simulink model "digital_twin_model_v2"  (R2023a)
settings: Solver=FixedStepAuto  StartTime=0.0  StopTime=515  FixedStep=ts  RelTol=1e-3
values from neighbouring files (symbols this model uses):
  Ccell0 = cell0 / v_cell    (= 15384.6153846)    [MainCode.m]
  CG0 = 185    [MainCode.m]
  cg_noGrowth = 10    [MainCode.m]
  CM = 4    [MainCode.m]
  CO0 = .245    (= 0.245)    [MainCode.m]
  count_thresh = 3    [MainCode.m]
  F_fresh_start = 5 * .016 * 60    (= 4.8)    [MainCode.m]
  F_net = F_fresh_start + F_recycle_start    (= 334.8)    [MainCode.m]
  F_recycle_start = 5 * 1.1 * 60    (= 330)    [MainCode.m]
  freshPump_response_increases = 2    [MainCode.m]
  freshPump_response_window = 10    [MainCode.m]
  g_fault_wait_time = 10    [MainCode.m]
  g_flowrate_control_windowsize = 10    [MainCode.m]
  g_lownoise_val = 1.25    [MainCode.m]
  g_numpoints_fail = g_standdev_window_size+1    (= 16)    [MainCode.m]
  g_numpoints_low = 4    [MainCode.m]
  g_prob_arraylen = 15    [MainCode.m]
  g_prob_count = 6    [MainCode.m]
  g_prob_thresh = .45    (= 0.45)    [MainCode.m]
  g_standdev_window_size = 15    [MainCode.m]
  g_standev_tol = 7    [MainCode.m]
  mu_max = 0.0251    [MainCode.m]
  n_size = t_window/ts    (= 2.5)    [MainCode.m]
  n_size_CG = n_size    (= 2.5)    [MainCode.m]
  o2_fail_mean = .008    (= 0.008)    [MainCode.m]
  o2_fault_halfrange = .01    (= 0.01)    [MainCode.m]
  o2_fault_numpoints = 5    [MainCode.m]
  o2_lownoise_val = .0008    (= 0.0008)    [MainCode.m]
  o2_numpoints_low = 6    [MainCode.m]
  o2_prob_arraylen = 10    [MainCode.m]
  o2_prob_count = 6    [MainCode.m]
  o2_prob_thresh = .45    (= 0.45)    [MainCode.m]
  OCR = 2.8e-11    [MainCode.m]
  p_thresh = .4    (= 0.4)    [MainCode.m]
  recPump_drop_val = .02    (= 0.02)    [MainCode.m]
  recPump_rollingavg_samples_buildup = 10    [MainCode.m]
  recPump_smallDrop_size = 0.006    [MainCode.m]
  t_crit_CG = .7    (= 0.7)    [MainCode.m]
  ts = 1    [MainCode.m]
  V = 65.0    (= 65)    [MainCode.m]
  v_cell = 65    [MainCode.m]
  YGC = 155 * 10^-6    (= 0.000155)    [MainCode.m]
undefined symbols (not defined in the file or in its folder): DiscIntNeverNeededParam
libraries: simulink x10, sldrtlib x9, dspstat3 x6, aerolibanimutils x1
(part 1 of 2)
settings Model: Creator=axtaw  LastModifiedBy=axtaw
settings ModelReferenceCC: ModelReferenceMinAlgLoopOccurrences=on

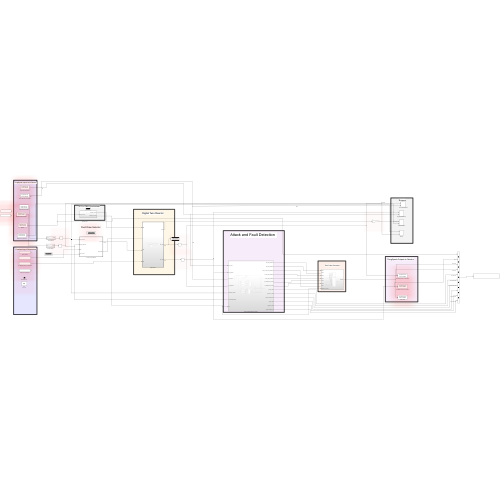
[thumbnail: Simulink's stored preview of the top-level diagram]
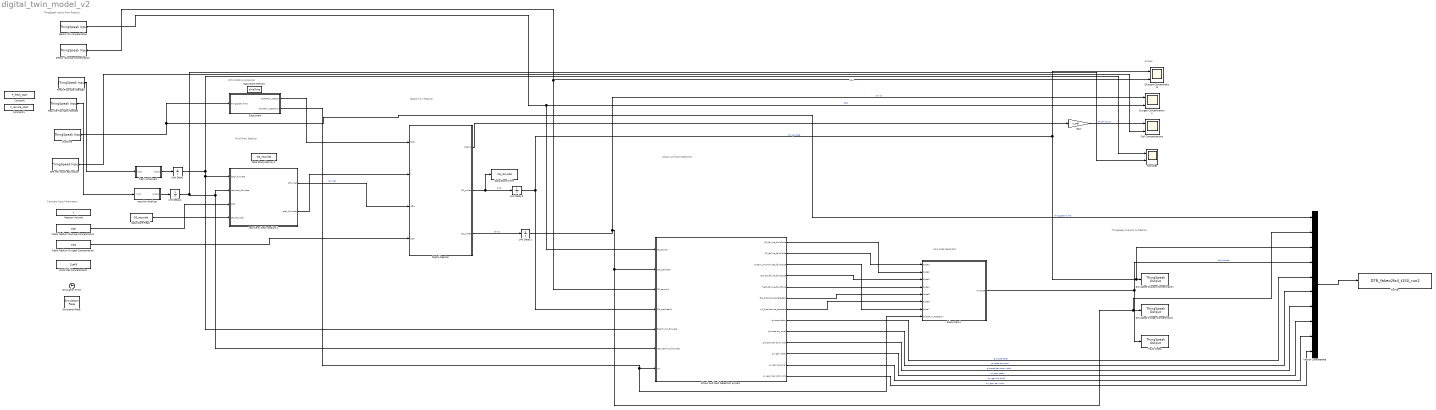
== system digital_twin_model_v2 ==
  note: Fluid Draw Selector
  note: DTR-CCBR Synchonizer
  note: Digital Twin Reactor
  note: Scopes
  note: Constant Input Parameters
  note: ThingSpeak Outputs to Reactor
  note: ThingSpeak Inputs from Reactor
  note: Attack and Fault Detection
  note: Faul Code Generator
  Attack and Fault Detection System : Subsystem
  Cell Concentrations : Scope  NumInputPorts=2
  Constant : Constant  Value=F_fresh_start
  Constant1 : Constant  Value=F_recycle_start
  Data Store Memory : DataStoreMemory  DataStoreName=aliveTime  WriteAfterWriteMsg=warning  ShowAdditionalParam=off
  Data Store Memory1 : DataStoreMemory  DataStoreName=CG_recycled  WriteAfterWriteMsg=warning  InitialValue=CG0  ShowAdditionalParam=off
  Data Store Read : DataStoreRead  DataStoreName=CG_recycled  IndexOptions=Index vector (dialog)  Indices=1  OutputSizes=1
  Data Store Write : DataStoreWrite  DataStoreName=CG_recycled  IndexOptions=Index vector (dialog)  Indices=1  OutputSizes=1
  Digital Reactor : Subsystem  TreatAsAtomicUnit=on
  Fault Codes : sldrtlib/Internet of Things/ThingSpeak Output  DrvAddress=2409205  DrvOptions=[1 1 50 75 54 78 55 57 69 50 79 79 81 55 79 66 88 72 97 112 105 46 116 104 105 110 103 115 112 101 97 107 46 99 111 109 0 0 0 0 0 0 0 0 0 0 0 0 0 0 0 0 0 0 0 0 0 0 0 0 0 0 0 0 0 0 0 0 0 0 0 0 0 0 0 0 0 0 0 0 0 0 0 0 0 0 0 0 0 0 0 0 0 0 0 0 0 0 0 0 0 0 0 0 0 0 0 0 0 0 0 0 0 0 0 0 0 0 0 0 0 0 0 0 0 0 0 0 0 0 0 0 0 0 0 0 0 0 0 0 0 0 0 0 0 0 0 0 0 0 0 0 0 0 0 0 0 0 0 0 0 0 0 0 0 0 0 0 0 0 0 0 0 0 0 0 0 0 0 0 0 0 0 0 0 0 0 0 0 0 0 0 0 0 0 0 0 0 0 0 0 0 0 0 0 0 0 0 0 0 0 0 0 0 0 0 0 0 0 0 0 0 0 0 0 0 0 0 0 0 0 0 0 0 0 0 0 0 0 0 0 0 0 0 0 0 0 0 0 0 0 0 0 0 0 0]  SampleTime=ts  MaxMissedTicks=1000  ShowMissedTicks=off  YieldWhenWaiting=off  ChannelFields=3  OptParam=0  InitialValue=[]  FinalValue=[]
  Fresh Flowrate Intended : sldrtlib/Internet of Things/ThingSpeak Input  DrvAddress=2409196  DrvOptions=[0 1 78 78 82 57 89 87 51 84 86 68 51 56 90 77 68 49 97 112 105 46 116 104 105 110 103 115 112 101 97 107 46 99 111 109 0 0 0 0 0 0 0 0 0 0 0 0 0 0 0 0 0 0 0 0 0 0 0 0 0 0 0 0 0 0 0 0 0 0 0 0 0 0 0 0 0 0 0 0 0 0 0 0 0 0 0 0 0 0 0 0 0 0 0 0 0 0 0 0 0 0 0 0 0 0 0 0 0 0 0 0 0 0 0 0 0 0 0 0 0 0 0 0 0 0 0 0 0 0 0 0 0 0 0 0 0 0 0 0 0 0 0 0 0 0 0 0 0 0 0 0 0 0 0 0 0 0 0 0 0 0 0 0 0 0 0 0 0 0 0 0 0 0 0 0 0 0 0 0 0 0 0 0 0 0 0 0 0 0 0 0 0 0 0 0 0 0 0 0 0 0 0 0 0 0 0 0 0 0 0 0 0 0 0 0 0 0 0 0 0 0 0 0 0 0 0 0 0 0 0 0 0 0 0 0 0 0 0 0 0 0 0 0 0 0 0 0 0 0 0 0 0 0 0 0]  SampleTime=ts  MaxMissedTicks=1000  ShowMissedTicks=off  YieldWhenWaiting=off  ChannelFields=3  OptParam=0  DataTypeStr=double
  Fresh Medium Glucose Concentration : Constant  Value=CG0
  Fresh Medium Oxygen Concentration : Constant  Value=CO0
  Gain : Gain  Gain=v_cell
  Glucose Concentrations : Scope  NumInputPorts=2
  Initial Cell Concentration : Constant  Value=Ccell0
  Oxygen Concentrations : Scope  NumInputPorts=2
  Reactor Volume : Constant  Value=V
  Recycle Flowrate Intended : sldrtlib/Internet of Things/ThingSpeak Input  DrvAddress=2409196  DrvOptions=[0 1 78 78 82 57 89 87 51 84 86 68 51 56 90 77 68 49 97 112 105 46 116 104 105 110 103 115 112 101 97 107 46 99 111 109 0 0 0 0 0 0 0 0 0 0 0 0 0 0 0 0 0 0 0 0 0 0 0 0 0 0 0 0 0 0 0 0 0 0 0 0 0 0 0 0 0 0 0 0 0 0 0 0 0 0 0 0 0 0 0 0 0 0 0 0 0 0 0 0 0 0 0 0 0 0 0 0 0 0 0 0 0 0 0 0 0 0 0 0 0 0 0 0 0 0 0 0 0 0 0 0 0 0 0 0 0 0 0 0 0 0 0 0 0 0 0 0 0 0 0 0 0 0 0 0 0 0 0 0 0 0 0 0 0 0 0 0 0 0 0 0 0 0 0 0 0 0 0 0 0 0 0 0 0 0 0 0 0 0 0 0 0 0 0 0 0 0 0 0 0 0 0 0 0 0 0 0 0 0 0 0 0 0 0 0 0 0 0 0 0 0 0 0 0 0 0 0 0 0 0 0 0 0 0 0 0 0 0 0 0 0 0 0 0 0 0 0 0 0 0 0 0 0 0 0]  SampleTime=ts  MaxMissedTicks=1000  ShowMissedTicks=off  YieldWhenWaiting=off  ChannelFields=2  OptParam=0  DataTypeStr=double
  Runtime : sldrtlib/Internet of Things/ThingSpeak Input  DrvAddress=2409196  DrvOptions=[0 1 78 78 82 57 89 87 51 84 86 68 51 56 90 77 68 49 97 112 105 46 116 104 105 110 103 115 112 101 97 107 46 99 111 109 0 0 0 0 0 0 0 0 0 0 0 0 0 0 0 0 0 0 0 0 0 0 0 0 0 0 0 0 0 0 0 0 0 0 0 0 0 0 0 0 0 0 0 0 0 0 0 0 0 0 0 0 0 0 0 0 0 0 0 0 0 0 0 0 0 0 0 0 0 0 0 0 0 0 0 0 0 0 0 0 0 0 0 0 0 0 0 0 0 0 0 0 0 0 0 0 0 0 0 0 0 0 0 0 0 0 0 0 0 0 0 0 0 0 0 0 0 0 0 0 0 0 0 0 0 0 0 0 0 0 0 0 0 0 0 0 0 0 0 0 0 0 0 0 0 0 0 0 0 0 0 0 0 0 0 0 0 0 0 0 0 0 0 0 0 0 0 0 0 0 0 0 0 0 0 0 0 0 0 0 0 0 0 0 0 0 0 0 0 0 0 0 0 0 0 0 0 0 0 0 0 0 0 0 0 0 0 0 0 0 0 0 0 0 0 0 0 0 0 0]  SampleTime=ts  MaxMissedTicks=1000  ShowMissedTicks=off  YieldWhenWaiting=off  ChannelFields=1  OptParam=0  DataTypeStr=double
  SPR cell count estimation : sldrtlib/Internet of Things/ThingSpeak Input  DrvAddress=2409196  DrvOptions=[0 1 78 78 82 57 89 87 51 84 86 68 51 56 90 77 68 49 97 112 105 46 116 104 105 110 103 115 112 101 97 107 46 99 111 109 0 0 0 0 0 0 0 0 0 0 0 0 0 0 0 0 0 0 0 0 0 0 0 0 0 0 0 0 0 0 0 0 0 0 0 0 0 0 0 0 0 0 0 0 0 0 0 0 0 0 0 0 0 0 0 0 0 0 0 0 0 0 0 0 0 0 0 0 0 0 0 0 0 0 0 0 0 0 0 0 0 0 0 0 0 0 0 0 0 0 0 0 0 0 0 0 0 0 0 0 0 0 0 0 0 0 0 0 0 0 0 0 0 0 0 0 0 0 0 0 0 0 0 0 0 0 0 0 0 0 0 0 0 0 0 0 0 0 0 0 0 0 0 0 0 0 0 0 0 0 0 0 0 0 0 0 0 0 0 0 0 0 0 0 0 0 0 0 0 0 0 0 0 0 0 0 0 0 0 0 0 0 0 0 0 0 0 0 0 0 0 0 0 0 0 0 0 0 0 0 0 0 0 0 0 0 0 0 0 0 0 0 0 0 0 0 0 0 0 0]  SampleTime=ts  MaxMissedTicks=1000  ShowMissedTicks=off  YieldWhenWaiting=off  ChannelFields=4  OptParam=0  DataTypeStr=double
  Sensor Glucose concentration : sldrtlib/Internet of Things/ThingSpeak Input  DrvAddress=2409196  DrvOptions=[0 1 78 78 82 57 89 87 51 84 86 68 51 56 90 77 68 49 97 112 105 46 116 104 105 110 103 115 112 101 97 107 46 99 111 109 0 0 0 0 0 0 0 0 0 0 0 0 0 0 0 0 0 0 0 0 0 0 0 0 0 0 0 0 0 0 0 0 0 0 0 0 0 0 0 0 0 0 0 0 0 0 0 0 0 0 0 0 0 0 0 0 0 0 0 0 0 0 0 0 0 0 0 0 0 0 0 0 0 0 0 0 0 0 0 0 0 0 0 0 0 0 0 0 0 0 0 0 0 0 0 0 0 0 0 0 0 0 0 0 0 0 0 0 0 0 0 0 0 0 0 0 0 0 0 0 0 0 0 0 0 0 0 0 0 0 0 0 0 0 0 0 0 0 0 0 0 0 0 0 0 0 0 0 0 0 0 0 0 0 0 0 0 0 0 0 0 0 0 0 0 0 0 0 0 0 0 0 0 0 0 0 0 0 0 0 0 0 0 0 0 0 0 0 0 0 0 0 0 0 0 0 0 0 0 0 0 0 0 0 0 0 0 0 0 0 0 0 0 0 0 0 0 0 0 0]  SampleTime=ts  MaxMissedTicks=1000  ShowMissedTicks=off  YieldWhenWaiting=off  ChannelFields=5  OptParam=0  DataTypeStr=double
  "Sensor O2 concentration " : sldrtlib/Internet of Things/ThingSpeak Input  DrvAddress=2409196  DrvOptions=[0 1 78 78 82 57 89 87 51 84 86 68 51 56 90 77 68 49 97 112 105 46 116 104 105 110 103 115 112 101 97 107 46 99 111 109 0 0 0 0 0 0 0 0 0 0 0 0 0 0 0 0 0 0 0 0 0 0 0 0 0 0 0 0 0 0 0 0 0 0 0 0 0 0 0 0 0 0 0 0 0 0 0 0 0 0 0 0 0 0 0 0 0 0 0 0 0 0 0 0 0 0 0 0 0 0 0 0 0 0 0 0 0 0 0 0 0 0 0 0 0 0 0 0 0 0 0 0 0 0 0 0 0 0 0 0 0 0 0 0 0 0 0 0 0 0 0 0 0 0 0 0 0 0 0 0 0 0 0 0 0 0 0 0 0 0 0 0 0 0 0 0 0 0 0 0 0 0 0 0 0 0 0 0 0 0 0 0 0 0 0 0 0 0 0 0 0 0 0 0 0 0 0 0 0 0 0 0 0 0 0 0 0 0 0 0 0 0 0 0 0 0 0 0 0 0 0 0 0 0 0 0 0 0 0 0 0 0 0 0 0 0 0 0 0 0 0 0 0 0 0 0 0 0 0 0]  SampleTime=ts  MaxMissedTicks=1000  ShowMissedTicks=off  YieldWhenWaiting=off  ChannelFields=6  OptParam=0  DataTypeStr=double
  Simulated Glucose Concentration : sldrtlib/Internet of Things/ThingSpeak Output  DrvAddress=2409205  DrvOptions=[1 1 50 75 54 78 55 57 69 50 79 79 81 55 79 66 88 72 97 112 105 46 116 104 105 110 103 115 112 101 97 107 46 99 111 109 0 0 0 0 0 0 0 0 0 0 0 0 0 0 0 0 0 0 0 0 0 0 0 0 0 0 0 0 0 0 0 0 0 0 0 0 0 0 0 0 0 0 0 0 0 0 0 0 0 0 0 0 0 0 0 0 0 0 0 0 0 0 0 0 0 0 0 0 0 0 0 0 0 0 0 0 0 0 0 0 0 0 0 0 0 0 0 0 0 0 0 0 0 0 0 0 0 0 0 0 0 0 0 0 0 0 0 0 0 0 0 0 0 0 0 0 0 0 0 0 0 0 0 0 0 0 0 0 0 0 0 0 0 0 0 0 0 0 0 0 0 0 0 0 0 0 0 0 0 0 0 0 0 0 0 0 0 0 0 0 0 0 0 0 0 0 0 0 0 0 0 0 0 0 0 0 0 0 0 0 0 0 0 0 0 0 0 0 0 0 0 0 0 0 0 0 0 0 0 0 0 0 0 0 0 0 0 0 0 0 0 0 0 0 0 0 0 0 0 0]  SampleTime=ts  MaxMissedTicks=1000  ShowMissedTicks=off  YieldWhenWaiting=off  ChannelFields=4  OptParam=0  InitialValue=[]  FinalValue=[]
  Simulated Oxygen Concentration : sldrtlib/Internet of Things/ThingSpeak Output  DrvAddress=2409205  DrvOptions=[1 1 50 75 54 78 55 57 69 50 79 79 81 55 79 66 88 72 97 112 105 46 116 104 105 110 103 115 112 101 97 107 46 99 111 109 0 0 0 0 0 0 0 0 0 0 0 0 0 0 0 0 0 0 0 0 0 0 0 0 0 0 0 0 0 0 0 0 0 0 0 0 0 0 0 0 0 0 0 0 0 0 0 0 0 0 0 0 0 0 0 0 0 0 0 0 0 0 0 0 0 0 0 0 0 0 0 0 0 0 0 0 0 0 0 0 0 0 0 0 0 0 0 0 0 0 0 0 0 0 0 0 0 0 0 0 0 0 0 0 0 0 0 0 0 0 0 0 0 0 0 0 0 0 0 0 0 0 0 0 0 0 0 0 0 0 0 0 0 0 0 0 0 0 0 0 0 0 0 0 0 0 0 0 0 0 0 0 0 0 0 0 0 0 0 0 0 0 0 0 0 0 0 0 0 0 0 0 0 0 0 0 0 0 0 0 0 0 0 0 0 0 0 0 0 0 0 0 0 0 0 0 0 0 0 0 0 0 0 0 0 0 0 0 0 0 0 0 0 0 0 0 0 0 0 0]  SampleTime=ts  MaxMissedTicks=1000  ShowMissedTicks=off  YieldWhenWaiting=off  ChannelFields=5  OptParam=0  InitialValue=[]  FinalValue=[]
  Simulation Pace : aerolibanimutils/Simulation Pace  SimulationPace=ts  SleepMode=Auto  OutputPaceError=off  SampleTime=ts
  Simulation Time : Clock
  Subsystem : Subsystem
  Subsystem1 : Subsystem
  To File : ToFile  Filename=DTR_fakeo2fail_t150_run2
  Unit Delay : UnitDelay  InitialCondition=F_fresh_start  SampleTime=-1  HasFrameUpgradeWarning=on
  Unit Delay1 : UnitDelay  InitialCondition=CO0  SampleTime=-1  HasFrameUpgradeWarning=on
  Unit Delay2 : UnitDelay  InitialCondition=F_recycle_start  SampleTime=-1  HasFrameUpgradeWarning=on
  Unit Delay3 : UnitDelay  InitialCondition=CG0  SampleTime=-1  HasFrameUpgradeWarning=on
  Vector Concatenate : Concatenate  NumInputs=10
  flowrates : Scope  NumInputPorts=2
  fresh initializer1 : Subsystem
  recycle initializer : Subsystem
  recycle or fresh medium1 : MATLAB Function  TreatAsAtomicUnit=on
  wires:
  recycle or fresh medium1/1(CG_inlet) -> Digital Reactor/3(CG0)  "cg inlet"
  recycle or fresh medium1/2(total_flowrate) -> Digital Reactor/2(F)
  Fresh Medium Oxygen Concentration/1 -> Digital Reactor/4(CO0)
  Fresh Medium Glucose Concentration/1 -> recycle or fresh medium1/3(CG0)
  Digital Reactor/1(CCell1) -> Gain/1
  Digital Reactor/3(CO_outlet) -> Unit Delay1/1  "dtr o2"
  Attack and Fault Detection System/2(O2_failure_faultCode) -> Subsystem1/1(Code1)
  Attack and Fault Detection System/4(recycle_failure_faultCode) -> Subsystem1/3(Code3)
  Attack and Fault Detection System/5(fresh_failure_faultCode) -> Subsystem1/4(Code4)
  Attack and Fault Detection System/1(GC_failure_faultCode) -> Subsystem1/2(Code2)
  Subsystem1/1(fullCode) -> Fault Codes/1, Vector Concatenate/4  "fault codes"
  Attack and Fault Detection System/6(GC_disturbance_detected) -> Subsystem1/5(Code5)
  Attack and Fault Detection System/7(o2_disturbance_detected) -> Subsystem1/6(Code6)
  Attack and Fault Detection System/3(system_ompromised_faultCode) -> Subsystem1/7(Code7)
  Vector Concatenate/1 -> To File/1
  Attack and Fault Detection System/8(glucose stdev) -> Vector Concatenate/5  "glucose stdev"
  Attack and Fault Detection System/9(glucose ab_small) -> Vector Concatenate/6  "glucose ab small"
  Attack and Fault Detection System/10(glucose deviation prob) -> Vector Concatenate/7  "glucose deviation prob"
  Attack and Fault Detection System/11(oxygen stdev) -> Vector Concatenate/8  "oxygen stdev"
  Attack and Fault Detection System/12(oxygen ab_small) -> Vector Concatenate/9  "oxygen ab small"
  Attack and Fault Detection System/13(oxygen deviation prob) -> Vector Concatenate/10  "oxygen dev prob"
  Gain/1 -> Cell Concentrations/1  "dtr cell count"
  Fresh Flowrate Intended/1 -> fresh initializer1/1(input)
  Recycle Flowrate Intended/1 -> recycle initializer/1(input)
  Runtime/1 -> Subsystem/1(thingspeak time), Vector Concatenate/1  "thingspeak time"
  Subsystem/1(doNotRun_reactor) -> Digital Reactor/1(DNR)
  SPR cell count estimation/1 -> Cell Concentrations/2
  Subsystem/2(doNotRun_detection) -> Subsystem1/8(doNotRun_detection), Attack and Fault Detection System/7(dnr)
  Digital Reactor/2(CG_outlet) -> Unit Delay3/1, Data Store Write/1  "DTR"
  Data Store Read/1 -> recycle or fresh medium1/4(CG_recycled)
  fresh initializer1/1(output) -> Unit Delay/1
  recycle initializer/1(output) -> Unit Delay2/1
  Unit Delay/1 -> Attack and Fault Detection System/5(freshPump_flowrate), recycle or fresh medium1/1(fresh_flowrate), flowrates/1
  Unit Delay2/1 -> recycle or fresh medium1/2(recycled_flowrate), Attack and Fault Detection System/6(recyclePump_flowrate), flowrates/2
  Sensor Glucose concentration/1 -> Glucose Concentrations/2, Attack and Fault Detection System/3(CG_sensor1)  "SPR"
  "Sensor O2 concentration "/1 -> Oxygen Concentrations/2, Attack and Fault Detection System/1(CO_sensor)  "SPR"
  Unit Delay1/1 -> Oxygen Concentrations/1, Vector Concatenate/2, Simulated Oxygen Concentration/1, Attack and Fault Detection System/2(CO_predicted)  "sim ox"
  Unit Delay3/1 -> Vector Concatenate/3, Simulated Glucose Concentration/1, Glucose Concentrations/1, Attack and Fault Detection System/4(CG_predicted1)  "sim glucose"

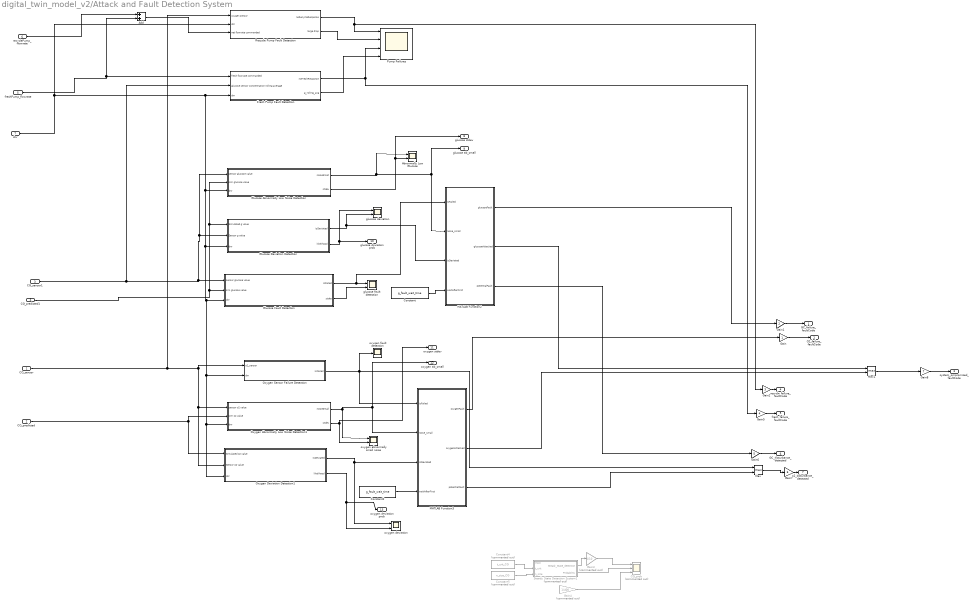
== system digital_twin_model_v2/Attack and Fault Detection System ==
  CO_sensor : Inport
  CO_predicted : Inport  Port=2
  CG_sensor1 : Inport  Port=3
  CG_predicted1 : Inport  Port=4
  freshPump_flowrate : Inport  Port=5
  recyclePump_flowrate : Inport  Port=6
  dnr : Inport  Port=7
  Abnormally Low Glucose : Scope  NumInputPorts=2
  Add : Sum
  CG_prob : Scope  Commented=on  NumInputPorts=3
  Constant : Constant  Value=g_fault_wait_time
  Constant2 : Constant  Value=g_fault_wait_time
  Constant4 : Constant  Commented=on  Value=t_crit_CG
  Constant5 : Constant  Commented=on  Value=n_size_CG
  Fresh Pump Fault Detection : Subsystem
  Gain : Gain
  Gain1 : Gain  Gain=2
  Gain2 : Gain  Gain=3
  Gain3 : Gain  Commented=on  Gain=1/10
  Gain4 : Gain  Commented=on  Gain=1/400
  Gain5 : Gain  Gain=4
  Gain6 : Gain  Gain=5
  Gain7 : Gain  Gain=6
  Gain8 : Gain  Gain=7
  Glucose Abnormally Low Noise Detection : Subsystem
  Glucose Deviation Detection : Subsystem
  Glucose Fault Detection : Subsystem
  MATLAB Function2 : MATLAB Function  TreatAsAtomicUnit=on
  MATLAB Function3 : MATLAB Function  TreatAsAtomicUnit=on
  Max : MinMax  Function=max  Inputs=2
  Max1 : MinMax  Function=max  Inputs=2
  Oxygen Abnormally Low Noise Detection1 : Subsystem
  Oxygen Deviation Detection1 : Subsystem
  Oxygen Sensor Failure Detection : Subsystem
  Pump Failures : Scope  NumInputPorts=4
  Recycle Pump Fault Detection : Subsystem
  Steady State Detection System1 : Subsystem  Commented=on
  glucose deviation : Scope  NumInputPorts=2
  glucose fault detection : Scope  NumInputPorts=2
  oxygen abnormally small noise : Scope  NumInputPorts=2
  oxygen deviation : Scope  NumInputPorts=2
  oxygen fault detection : Scope
  GC_failure_faultCode : Outport
  O2_failure_faultCode : Outport  Port=2
  system_ompromised_faultCode : Outport  Port=3
  recycle_failure_faultCode : Outport  Port=4
  fresh_failure_faultCode : Outport  Port=5
  GC_disturbance_detected : Outport  Port=6
  o2_disturbance_detected : Outport  Port=7
  glucose stdev : Outport  Port=8
  glucose ab_small : Outport  Port=9
  glucose deviation prob : Outport  Port=10
  oxygen stdev : Outport  Port=11
  oxygen ab_small : Outport  Port=12
  oxygen deviation prob : Outport  Port=13
  wires:
  CO_sensor/1 -> Recycle Pump Fault Detection/1(oxygen sensor), Oxygen Deviation Detection1/2(Sensor o2 value), Oxygen Abnormally Low Noise Detection1/1(sensor o2 value), Oxygen Sensor Failure Detection/1(o2_sensor)
  CG_sensor1/1 -> Fresh Pump Fault Detection/2(glucose sensor concentration rolling average), Glucose Abnormally Low Noise Detection/1(sensor glucose value), Glucose Deviation Detection/2(Sensor g value), Glucose Fault Detection/1(sensor glucose value)
  CG_predicted1/1 -> Glucose Abnormally Low Noise Detection/2(sim glucose value), Glucose Deviation Detection/1(Simulated g value), Glucose Fault Detection/2(sim glucose value)
  Gain4/1 -> CG_prob/3
  Gain3/1 -> CG_prob/1
  Constant4/1 -> Steady State Detection System1/2(t_crit)
  Steady State Detection System1/1(Steady_State_detection) -> Gain3/1
  Constant5/1 -> Steady State Detection System1/3(n_size)
  Steady State Detection System1/2(Probability) -> CG_prob/2
  CO_predicted/1 -> Oxygen Deviation Detection1/1(Simulated o2 value), Oxygen Abnormally Low Noise Detection1/2(sim o2 value)
  Glucose Abnormally Low Noise Detection/1(noiseSmall) -> Abnormally Low Glucose/1, glucose ab_small/1, MATLAB Function2/2(noise_small)
  Glucose Deviation Detection/1(isDeviated) -> glucose deviation/2, MATLAB Function2/3(isDeviated)
  Glucose Fault Detection/1(isFailed) -> MATLAB Function2/1(isFailed), glucose fault detection/1
  Constant/1 -> MATLAB Function2/4(waitAfterFirst)
  MATLAB Function2/3(potentialFault) -> Gain6/1
  MATLAB Function2/2(glucoseAttacked) -> Max1/1
  MATLAB Function2/1(glucoseFault) -> Gain1/1
  Glucose Abnormally Low Noise Detection/2(stdev) -> glucose stdev/1, Abnormally Low Glucose/2
  Constant2/1 -> MATLAB Function3/4(waitAfterFirst)
  Oxygen Sensor Failure Detection/1(isFailed) -> Max/1, oxygen fault detection/1, MATLAB Function3/1(isFailed)
  Oxygen Abnormally Low Noise Detection1/1(noiseSmall) -> MATLAB Function3/2(noise_small), oxygen ab_small/1, oxygen abnormally small noise/1
  Oxygen Deviation Detection1/1(isDeviated) -> MATLAB Function3/3(isDeviated), oxygen deviation/1
  Oxygen Abnormally Low Noise Detection1/2(stdev) -> oxygen stdev/1, oxygen abnormally small noise/2
  Oxygen Deviation Detection1/2(likelihood) -> oxygen deviation prob/1, oxygen deviation/2
  MATLAB Function3/3(potentialFault) -> Max/2
  MATLAB Function3/2(oxygenAttacked) -> Max1/2
  MATLAB Function3/1(oxygenFault) -> Gain/1
  freshPump_flowrate/1 -> Add/2, Fresh Pump Fault Detection/1(fresh flowrate commanded)
  Fresh Pump Fault Detection/1(noFreshResponse) -> Gain5/1, Pump Failures/3
  Glucose Deviation Detection/2(likelihood) -> glucose deviation prob/1, glucose deviation/1
  Glucose Fault Detection/2(stdev) -> glucose fault detection/2
  recyclePump_flowrate/1 -> Add/1
  Add/1 -> Recycle Pump Fault Detection/3(net flowrate commanded)
  Recycle Pump Fault Detection/1(noRecycleResponse) -> Pump Failures/1, Gain2/1
  Max1/1 -> Gain8/1
  Max/1 -> Gain7/1
  dnr/1 -> Oxygen Deviation Detection1/3(dnr), Oxygen Abnormally Low Noise Detection1/3(dnr), Oxygen Sensor Failure Detection/2(dnr), Glucose Fault Detection/3(dnr), Glucose Deviation Detection/3(dnr), Glucose Abnormally Low Noise Detection/3(dnr), Fresh Pump Fault Detection/3(dnr), Recycle Pump Fault Detection/2(dnr)
  Gain/1 -> O2_failure_faultCode/1
  Gain1/1 -> GC_failure_faultCode/1
  Gain2/1 -> recycle_failure_faultCode/1
  Gain5/1 -> fresh_failure_faultCode/1
  Gain6/1 -> GC_disturbance_detected/1
  Gain7/1 -> o2_disturbance_detected/1
  Gain8/1 -> system_ompromised_faultCode/1
  Fresh Pump Fault Detection/2(g_rolling_avg) -> Pump Failures/4
  Recycle Pump Fault Detection/2(large drop) -> Pump Failures/2

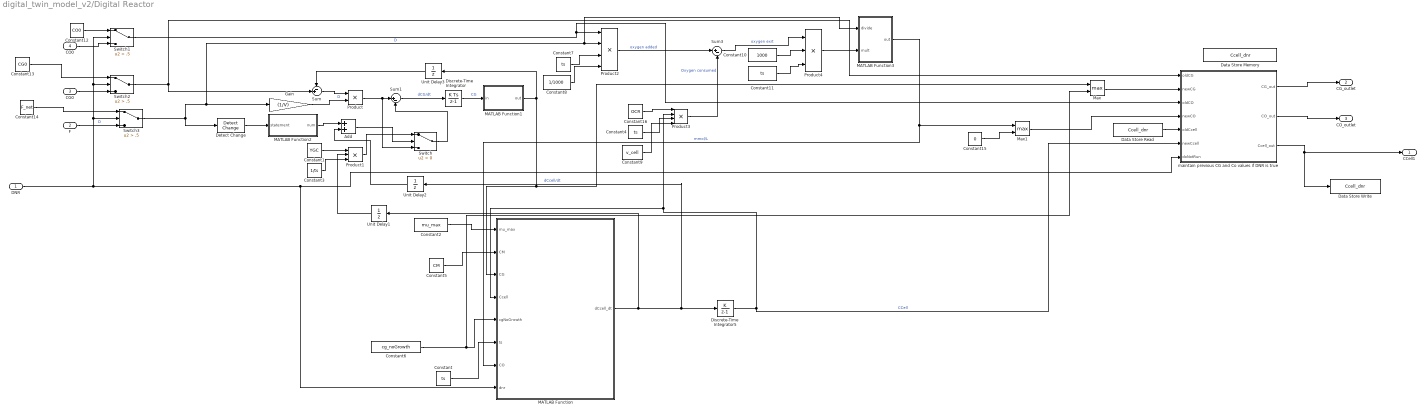
== system digital_twin_model_v2/Digital Reactor ==
  DNR : Inport
  F : Inport  Port=2
  CG0 : Inport  Port=3
  CO0 : Inport  Port=4
  Add : Sum
  Constant{,4,7,11} (4 alike) : Constant  Value=ts
  Constant1 : Constant  Value=YGC
  Constant10 : Constant  Value=1000
  Constant12 : Constant  Value=CO0
  Constant13 : Constant  Value=CG0
  Constant14 : Constant  Value=F_net
  Constant15 : Constant  Value=0
  Constant16 : Constant  Value=OCR
  Constant2 : Constant  Value=mu_max
  Constant3 : Constant  Value=1/ts
  Constant5 : Constant  Value=CM
  Constant6 : Constant  Value=cg_noGrowth
  Constant8 : Constant  Value=1/1000
  Constant9 : Constant  Value=v_cell
  Data Store Memory : DataStoreMemory  DataStoreName=Ccell_dnr  WriteAfterWriteMsg=warning  InitialValue=Ccell0  ShowAdditionalParam=off
  Data Store Read : DataStoreRead  DataStoreName=Ccell_dnr  IndexOptions=Index vector (dialog)  Indices=1  OutputSizes=1
  Data Store Write : DataStoreWrite  DataStoreName=Ccell_dnr  IndexOptions=Index vector (dialog)  Indices=1  OutputSizes=1
  Detect Change : simulink/Logic and Bit Operations/Detect Change  vinit=0  OutDataTypeStr=boolean
  Discrete-Time Integrator : DiscreteIntegrator  Priority=0  InitialCondition=CG0  SampleTime=ts  ICPrevOutput=DiscIntNeverNeededParam  ICPrevScaledInput=DiscIntNeverNeededParam
  Discrete-Time Integrator5 : DiscreteIntegrator  IntegratorMethod=Accumulation: Forward Euler  InitialCondition=Ccell0  SampleTime=ts  ICPrevOutput=DiscIntNeverNeededParam  ICPrevScaledInput=DiscIntNeverNeededParam
  Gain : Gain  Gain=(1/V)
  MATLAB Function : MATLAB Function  Priority=0  TreatAsAtomicUnit=on
  MATLAB Function1 : MATLAB Function  TreatAsAtomicUnit=on
  MATLAB Function2 : MATLAB Function  TreatAsAtomicUnit=on
  MATLAB Function3 : MATLAB Function  TreatAsAtomicUnit=on
  Max : MinMax  Function=max  Inputs=2
  Max1 : MinMax  Function=max  Inputs=2
  Product : Product
  Product1 : Product  Inputs=3
  Product2 : Product  Inputs=4
  Product3 : Product  Inputs=4
  Product4 : Product  Inputs=3
  Sum : Sum  Inputs=-+|
  Sum1 : Sum  Inputs=|+-
  Sum3 : Sum  Inputs=|+-
  Switch : Switch  Criteria=u2 > Threshold  SaturateOnIntegerOverflow=off  InputSameDT=off
  Switch1 : Switch  Criteria=u2 > Threshold  Threshold=.5  SaturateOnIntegerOverflow=off  InputSameDT=off
  Switch2 : Switch  Criteria=u2 > Threshold  Threshold=.5  SaturateOnIntegerOverflow=off  InputSameDT=off
  Switch3 : Switch  Criteria=u2 > Threshold  Threshold=.5  SaturateOnIntegerOverflow=off  InputSameDT=off
  Unit Delay1 : UnitDelay  SampleTime=-1  HasFrameUpgradeWarning=on
  Unit Delay2 : UnitDelay  SampleTime=-1  HasFrameUpgradeWarning=on
  Unit Delay3 : UnitDelay  InitialCondition=CG0  SampleTime=-1  HasFrameUpgradeWarning=on
  maintain previous CG and Co values if DNR is true : MATLAB Function  TreatAsAtomicUnit=on
  CCell1 : Outport
  CG_outlet : Outport  Port=2
  CO_outlet : Outport  Port=3
  wires:
  Data Store Read/1 -> maintain previous CG and Co values if DNR is true/5(oldCcell)
  Switch1/1 -> maintain previous CG and Co values if DNR is true/3(oldCO), Product2/1
  MATLAB Function3/1(out) -> Max1/1, MATLAB Function/7(CO)  "mmol/L"
  MATLAB Function2/1(num) -> Add/1
  Product4/1 -> MATLAB Function3/2(mult)
  Sum/1 -> Product/1
  Switch2/1 -> maintain previous CG and Co values if DNR is true/1(oldCG), Sum/2
  Constant7/1 -> Product2/3
  Constant4/1 -> Product3/3
  Constant2/1 -> MATLAB Function/1(mu_max)
  Constant6/1 -> Max/2, MATLAB Function/5(cgNoGrowth)
  Constant1/1 -> Product1/1
  Product2/1 -> Sum3/1  "oxygen added"
  Constant8/1 -> Product2/4
  Constant/1 -> MATLAB Function/6(ts)
  Constant16/1 -> Product3/1
  Switch3/1 -> MATLAB Function3/1(divide), Product2/2, Gain/1, Detect Change/1  "D"
  Product1/1 -> Switch/1
  Discrete-Time Integrator/1 -> MATLAB Function1/1(in)  "CG"
  Sum3/1 -> Product4/1  "oxygen exit"
  Constant10/1 -> Product4/2
  Add/1 -> Switch/2
  MATLAB Function/1(dCcell_dt) -> Discrete-Time Integrator5/1, Unit Delay2/1, Unit Delay1/1  "dCcell/dt"
  Gain/1 -> Product/2  "D"
  Constant3/1 -> Product1/3
  Constant11/1 -> Product4/3
  Discrete-Time Integrator5/1 -> maintain previous CG and Co values if DNR is true/6(newCcell), Product3/2, MATLAB Function/4(Ccell)  "CCell"
  Constant5/1 -> MATLAB Function/2(CM)
  Detect Change/1 -> MATLAB Function2/1(statement)
  Sum1/1 -> Discrete-Time Integrator/1  "dCG/dt"
  Product3/1 -> Sum3/2  "Oxygen consumed"
  Constant9/1 -> Product3/4
  Product/1 -> Switch/3, Sum1/1
  DNR/1 -> Switch1/2, Switch2/2, Switch3/2, MATLAB Function/8(dnr), maintain previous CG and Co values if DNR is true/7(doNotRun)
  maintain previous CG and Co values if DNR is true/3(Ccell_out) -> Data Store Write/1, CCell1/1
  maintain previous CG and Co values if DNR is true/2(CO_out) -> CO_outlet/1
  maintain previous CG and Co values if DNR is true/1(CG_out) -> CG_outlet/1
  Switch/1 -> Sum1/2
  CO0/1 -> Switch1/3
  CG0/1 -> Switch2/3
  F/1 -> Switch3/3  "D"
  Constant12/1 -> Switch1/1
  Constant13/1 -> Switch2/1
  Constant14/1 -> Switch3/1
  Unit Delay2/1 -> Add/2
  Unit Delay1/1 -> Product1/2
  MATLAB Function1/1(out) -> Max/1, MATLAB Function/3(CG), Unit Delay3/1
  Unit Delay3/1 -> Sum/1
  Max/1 -> maintain previous CG and Co values if DNR is true/2(newCG)
  Max1/1 -> maintain previous CG and Co values if DNR is true/4(newCO)
  Constant15/1 -> Max1/2

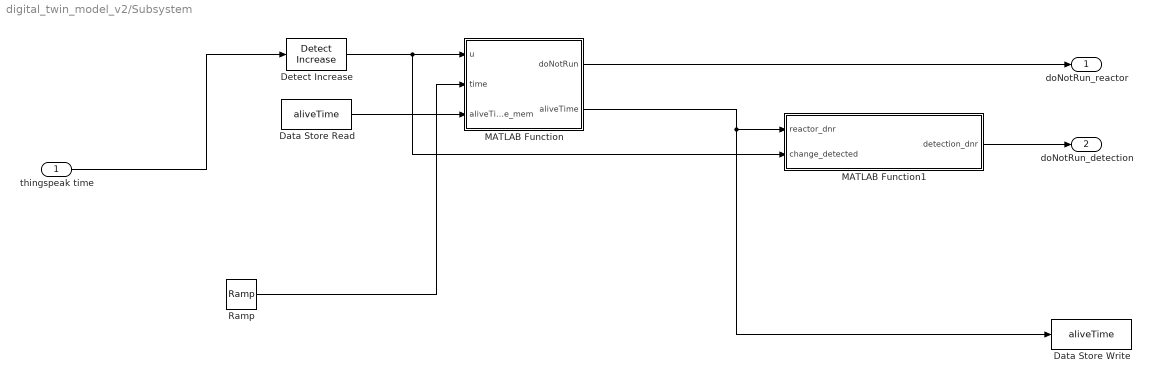
== system digital_twin_model_v2/Subsystem ==
  thingspeak time : Inport
  Data Store Read : DataStoreRead  DataStoreName=aliveTime  IndexOptions=Index vector (dialog)  Indices=1  OutputSizes=1
  Data Store Write : DataStoreWrite  DataStoreName=aliveTime  IndexOptions=Index vector (dialog)  Indices=1  OutputSizes=1
  Detect Increase : simulink/Logic and Bit Operations/Detect Increase  vinit=9999  OutDataTypeStr=boolean
  MATLAB Function : MATLAB Function  TreatAsAtomicUnit=on
  MATLAB Function1 : MATLAB Function  TreatAsAtomicUnit=on
  Ramp : simulink/Sources/Ramp  slope=1  start=0  InitialOutput=0
  doNotRun_reactor : Outport
  doNotRun_detection : Outport  Port=2
  wires:
  MATLAB Function/1(doNotRun) -> doNotRun_reactor/1
  Detect Increase/1 -> MATLAB Function1/2(change_detected), MATLAB Function/1(u)
  thingspeak time/1 -> Detect Increase/1
  Ramp/1 -> MATLAB Function/2(time)
  MATLAB Function/2(aliveTime) -> Data Store Write/1, MATLAB Function1/1(reactor_dnr)
  Data Store Read/1 -> MATLAB Function/3(aliveTime_mem)
  MATLAB Function1/1(detection_dnr) -> doNotRun_detection/1

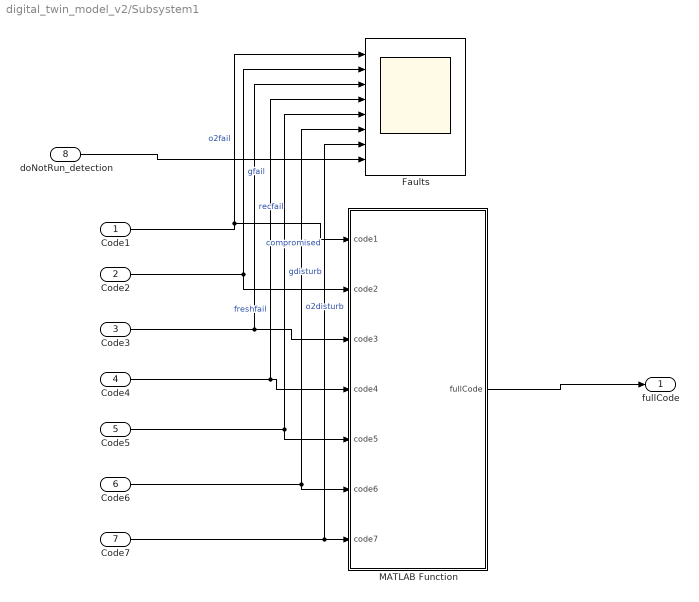
== system digital_twin_model_v2/Subsystem1 ==
  Code1 : Inport
  Code2 : Inport  Port=2
  Code3 : Inport  Port=3
  Code4 : Inport  Port=4
  Code5 : Inport  Port=5
  Code6 : Inport  Port=6
  Code7 : Inport  Port=7
  doNotRun_detection : Inport  Port=8
  Faults : Scope  NumInputPorts=8
  MATLAB Function : MATLAB Function  TreatAsAtomicUnit=on
  fullCode : Outport
  wires:
  Code1/1 -> Faults/1, MATLAB Function/1(code1)  "o2fail"
  MATLAB Function/1(fullCode) -> fullCode/1
  Code2/1 -> MATLAB Function/2(code2), Faults/2  "gfail"
  Code3/1 -> Faults/3, MATLAB Function/3(code3)  "recfail"
  Code4/1 -> Faults/4, MATLAB Function/4(code4)  "freshfail"
  Code5/1 -> MATLAB Function/5(code5), Faults/5  "gdisturb"
  Code6/1 -> MATLAB Function/6(code6), Faults/6  "o2disturb"
  Code7/1 -> Faults/7, MATLAB Function/7(code7)  "compromised"
  doNotRun_detection/1 -> Faults/8

== system digital_twin_model_v2/fresh initializer1 ==
  input : Inport
  Constant : Constant  Value=F_fresh_start
  MATLAB Function : MATLAB Function  TreatAsAtomicUnit=on
  Ramp : simulink/Sources/Ramp  slope=1  start=0  InitialOutput=0
  output : Outport
  wires:
  MATLAB Function/1(output) -> output/1
  input/1 -> MATLAB Function/1(input)
  Ramp/1 -> MATLAB Function/3(time)
  Constant/1 -> MATLAB Function/2(initial_val)

== system digital_twin_model_v2/recycle initializer ==
  input : Inport
  Constant : Constant  Value=F_recycle_start
  MATLAB Function : MATLAB Function  TreatAsAtomicUnit=on
  Ramp : simulink/Sources/Ramp  slope=1  start=0  InitialOutput=0
  output : Outport
  wires:
  MATLAB Function/1(output) -> output/1
  input/1 -> MATLAB Function/1(input)
  Ramp/1 -> MATLAB Function/3(time)
  Constant/1 -> MATLAB Function/2(initial_val)

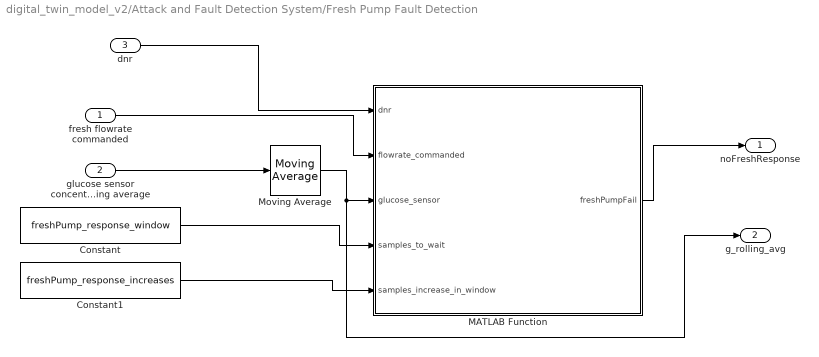
== system digital_twin_model_v2/Attack and Fault Detection System/Fresh Pump Fault Detection ==
  fresh flowrate commanded : Inport
  glucose sensor concentration rolling average : Inport  Port=2
  dnr : Inport  Port=3
  Constant : Constant  Value=freshPump_response_window
  Constant1 : Constant  Value=freshPump_response_increases
  MATLAB Function : MATLAB Function  TreatAsAtomicUnit=on
  Moving Average : dspstat3/Moving Average  Method=Sliding window  ForgettingFactorPort=off  SpecifyWindowLength=on  WindowLength=g_flowrate_control_windowsize  OverlapLength=g_flowrate_control_windowsize-1  AllowArbitraryInputLength=off  ForgettingFactor=0.9  SimulateUsing=Code generation
  noFreshResponse : Outport
  g_rolling_avg : Outport  Port=2
  wires:
  glucose sensor concentration rolling average/1 -> Moving Average/1
  fresh flowrate commanded/1 -> MATLAB Function/2(flowrate_commanded)
  Constant/1 -> MATLAB Function/4(samples_to_wait)
  Constant1/1 -> MATLAB Function/5(samples_increase_in_window)
  MATLAB Function/1(freshPumpFail) -> noFreshResponse/1
  Moving Average/1 -> g_rolling_avg/1, MATLAB Function/3(glucose_sensor)
  dnr/1 -> MATLAB Function/1(dnr)

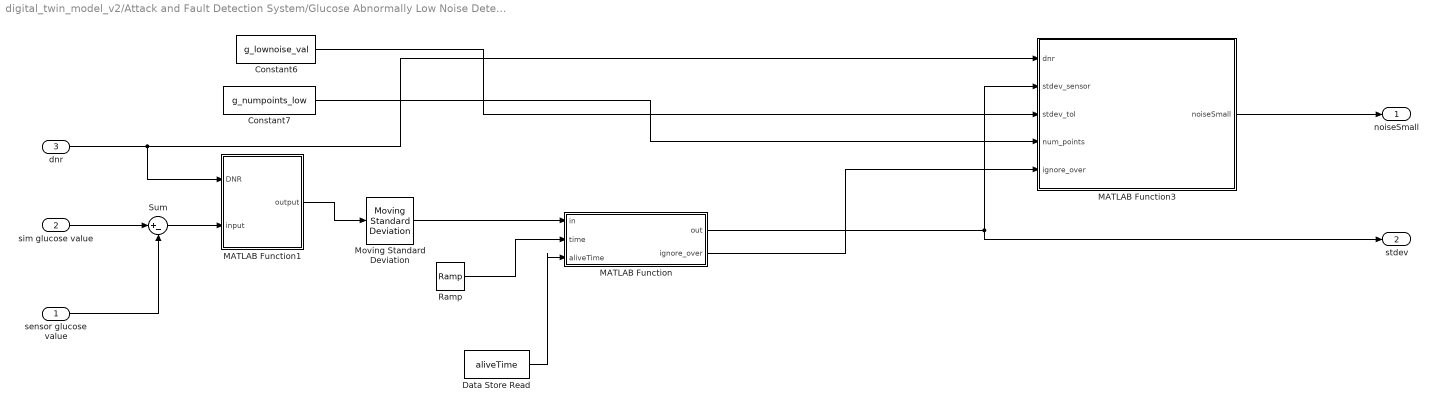
== system digital_twin_model_v2/Attack and Fault Detection System/Glucose Abnormally Low Noise Detection ==
  sensor glucose value : Inport
  sim glucose value : Inport  Port=2
  dnr : Inport  Port=3
  Constant6 : Constant  Value=g_lownoise_val
  Constant7 : Constant  Value=g_numpoints_low
  Data Store Read : DataStoreRead  DataStoreName=aliveTime  IndexOptions=Index vector (dialog)  Indices=1  OutputSizes=1
  MATLAB Function : MATLAB Function  TreatAsAtomicUnit=on
  MATLAB Function1 : MATLAB Function  TreatAsAtomicUnit=on
  MATLAB Function3 : MATLAB Function  TreatAsAtomicUnit=on
  Moving Standard Deviation : dspstat3/Moving Standard Deviation  Method=Sliding window  ForgettingFactorPort=off  SpecifyWindowLength=on  WindowLength=g_standdev_window_size  OverlapLength=g_standdev_window_size-1  AllowArbitraryInputLength=off  ForgettingFactor=0.9  SimulateUsing=Code generation
  Ramp : simulink/Sources/Ramp  slope=1  start=0  InitialOutput=0
  Sum : Sum  Inputs=|+-
  noiseSmall : Outport
  stdev : Outport  Port=2
  wires:
  MATLAB Function3/1(noiseSmall) -> noiseSmall/1
  Sum/1 -> MATLAB Function1/2(input)
  Moving Standard Deviation/1 -> MATLAB Function/1(in)
  Ramp/1 -> MATLAB Function/2(time)
  sim glucose value/1 -> Sum/1
  MATLAB Function/1(out) -> MATLAB Function3/2(stdev_sensor), stdev/1
  sensor glucose value/1 -> Sum/2
  Constant6/1 -> MATLAB Function3/3(stdev_tol)
  Constant7/1 -> MATLAB Function3/4(num_points)
  MATLAB Function/2(ignore_over) -> MATLAB Function3/5(ignore_over)
  dnr/1 -> MATLAB Function1/1(DNR), MATLAB Function3/1(dnr)
  Data Store Read/1 -> MATLAB Function/3(aliveTime)
  MATLAB Function1/1(output) -> Moving Standard Deviation/1

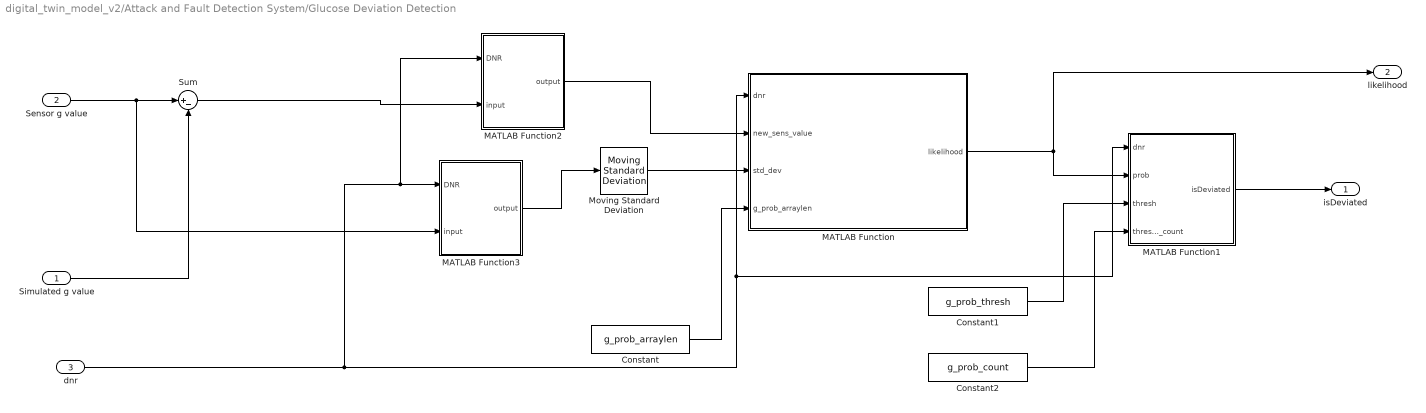
== system digital_twin_model_v2/Attack and Fault Detection System/Glucose Deviation Detection ==
  Simulated g value : Inport
  Sensor g value : Inport  Port=2
  dnr : Inport  Port=3
  Constant : Constant  Value=g_prob_arraylen
  Constant1 : Constant  Value=g_prob_thresh
  Constant2 : Constant  Value=g_prob_count
  MATLAB Function : MATLAB Function  TreatAsAtomicUnit=on
  MATLAB Function1 : MATLAB Function  TreatAsAtomicUnit=on
  MATLAB Function2 : MATLAB Function  TreatAsAtomicUnit=on
  MATLAB Function3 : MATLAB Function  TreatAsAtomicUnit=on
  Moving Standard Deviation : dspstat3/Moving Standard Deviation  Method=Sliding window  ForgettingFactorPort=off  SpecifyWindowLength=on  WindowLength=g_standdev_window_size  OverlapLength=g_standdev_window_size-1  AllowArbitraryInputLength=off  ForgettingFactor=0.9  SimulateUsing=Code generation
  Sum : Sum  Inputs=|+-
  isDeviated : Outport
  likelihood : Outport  Port=2
  wires:
  Moving Standard Deviation/1 -> MATLAB Function/3(std_dev)
  MATLAB Function/1(likelihood) -> likelihood/1, MATLAB Function1/2(prob)
  Simulated g value/1 -> Sum/2
  Constant/1 -> MATLAB Function/4(g_prob_arraylen)
  Sensor g value/1 -> MATLAB Function3/2(input), Sum/1
  Sum/1 -> MATLAB Function2/2(input)
  MATLAB Function1/1(isDeviated) -> isDeviated/1
  Constant1/1 -> MATLAB Function1/3(thresh)
  Constant2/1 -> MATLAB Function1/4(thresh_count)
  dnr/1 -> MATLAB Function2/1(DNR), MATLAB Function3/1(DNR), MATLAB Function1/1(dnr), MATLAB Function/1(dnr)
  MATLAB Function2/1(output) -> MATLAB Function/2(new_sens_value)
  MATLAB Function3/1(output) -> Moving Standard Deviation/1

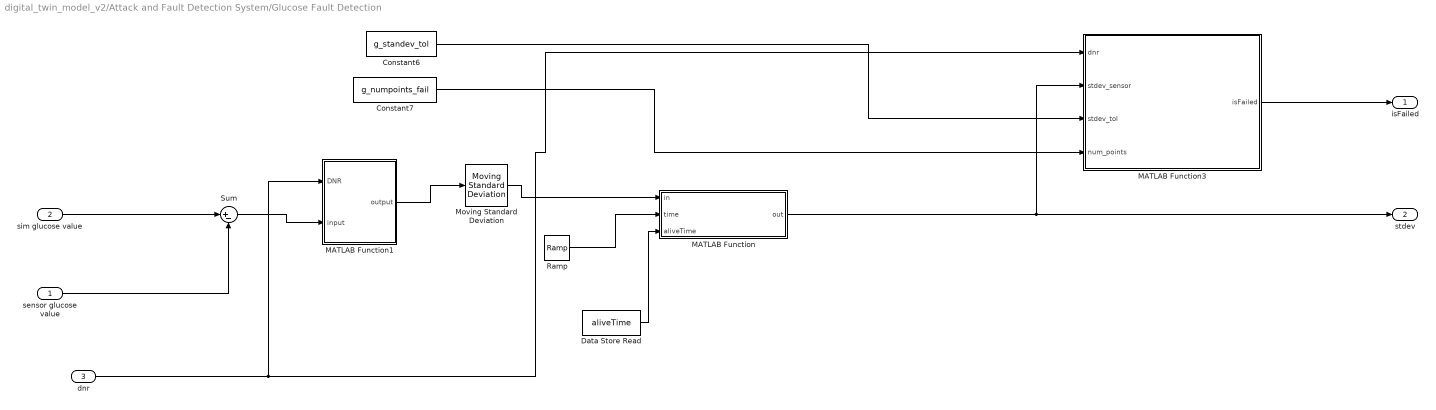
== system digital_twin_model_v2/Attack and Fault Detection System/Glucose Fault Detection ==
  sensor glucose value : Inport
  sim glucose value : Inport  Port=2
  dnr : Inport  Port=3
  Constant6 : Constant  Value=g_standev_tol
  Constant7 : Constant  Value=g_numpoints_fail
  Data Store Read : DataStoreRead  DataStoreName=aliveTime  IndexOptions=Index vector (dialog)  Indices=1  OutputSizes=1
  MATLAB Function : MATLAB Function  TreatAsAtomicUnit=on
  MATLAB Function1 : MATLAB Function  TreatAsAtomicUnit=on
  MATLAB Function3 : MATLAB Function  TreatAsAtomicUnit=on
  Moving Standard Deviation : dspstat3/Moving Standard Deviation  Method=Sliding window  ForgettingFactorPort=off  SpecifyWindowLength=on  WindowLength=g_standdev_window_size  OverlapLength=g_standdev_window_size-1  AllowArbitraryInputLength=off  ForgettingFactor=0.9  SimulateUsing=Code generation
  Ramp : simulink/Sources/Ramp  slope=1  start=0  InitialOutput=0
  Sum : Sum  Inputs=|+-
  isFailed : Outport
  stdev : Outport  Port=2
  wires:
  sim glucose value/1 -> Sum/1
  sensor glucose value/1 -> Sum/2
  MATLAB Function/1(out) -> stdev/1, MATLAB Function3/2(stdev_sensor)
  Sum/1 -> MATLAB Function1/2(input)
  Moving Standard Deviation/1 -> MATLAB Function/1(in)
  Constant7/1 -> MATLAB Function3/4(num_points)
  Constant6/1 -> MATLAB Function3/3(stdev_tol)
  Ramp/1 -> MATLAB Function/2(time)
  MATLAB Function3/1(isFailed) -> isFailed/1
  dnr/1 -> MATLAB Function3/1(dnr), MATLAB Function1/1(DNR)
  Data Store Read/1 -> MATLAB Function/3(aliveTime)
  MATLAB Function1/1(output) -> Moving Standard Deviation/1

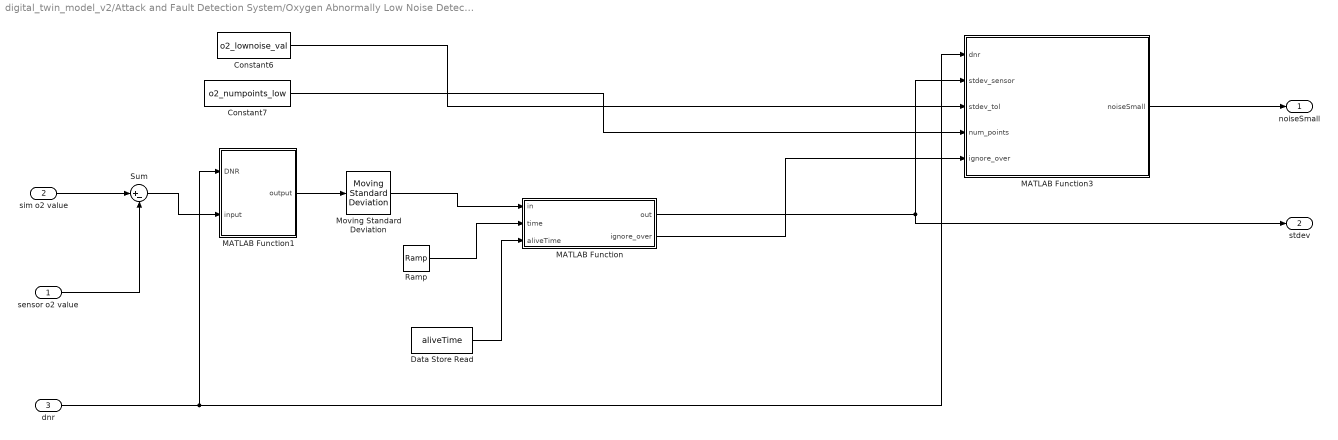
== system digital_twin_model_v2/Attack and Fault Detection System/Oxygen Abnormally Low Noise Detection1 ==
  sensor o2 value : Inport
  sim o2 value : Inport  Port=2
  dnr : Inport  Port=3
  Constant6 : Constant  Value=o2_lownoise_val
  Constant7 : Constant  Value=o2_numpoints_low
  Data Store Read : DataStoreRead  DataStoreName=aliveTime  IndexOptions=Index vector (dialog)  Indices=1  OutputSizes=1
  MATLAB Function : MATLAB Function  TreatAsAtomicUnit=on
  MATLAB Function1 : MATLAB Function  TreatAsAtomicUnit=on
  MATLAB Function3 : MATLAB Function  TreatAsAtomicUnit=on
  Moving Standard Deviation : dspstat3/Moving Standard Deviation  Method=Sliding window  ForgettingFactorPort=off  SpecifyWindowLength=on  WindowLength=g_standdev_window_size  OverlapLength=g_standdev_window_size-1  AllowArbitraryInputLength=off  ForgettingFactor=0.9  SimulateUsing=Code generation
  Ramp : simulink/Sources/Ramp  slope=1  start=0  InitialOutput=0
  Sum : Sum  Inputs=|+-
  noiseSmall : Outport
  stdev : Outport  Port=2
  wires:
  MATLAB Function3/1(noiseSmall) -> noiseSmall/1
  Sum/1 -> MATLAB Function1/2(input)
  Moving Standard Deviation/1 -> MATLAB Function/1(in)
  Ramp/1 -> MATLAB Function/2(time)
  sim o2 value/1 -> Sum/1
  MATLAB Function/1(out) -> MATLAB Function3/2(stdev_sensor), stdev/1
  sensor o2 value/1 -> Sum/2
  Constant6/1 -> MATLAB Function3/3(stdev_tol)
  Constant7/1 -> MATLAB Function3/4(num_points)
  MATLAB Function/2(ignore_over) -> MATLAB Function3/5(ignore_over)
  dnr/1 -> MATLAB Function1/1(DNR), MATLAB Function3/1(dnr)
  Data Store Read/1 -> MATLAB Function/3(aliveTime)
  MATLAB Function1/1(output) -> Moving Standard Deviation/1

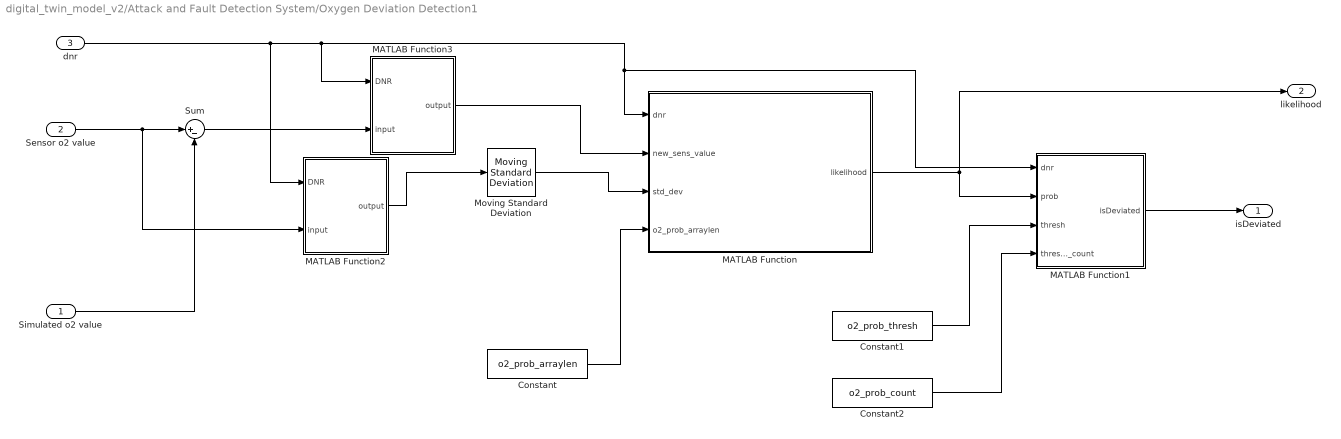
== system digital_twin_model_v2/Attack and Fault Detection System/Oxygen Deviation Detection1 ==
  Simulated o2 value : Inport
  Sensor o2 value : Inport  Port=2
  dnr : Inport  Port=3
  Constant : Constant  Value=o2_prob_arraylen
  Constant1 : Constant  Value=o2_prob_thresh
  Constant2 : Constant  Value=o2_prob_count
  MATLAB Function : MATLAB Function  TreatAsAtomicUnit=on
  MATLAB Function1 : MATLAB Function  TreatAsAtomicUnit=on
  MATLAB Function2 : MATLAB Function  TreatAsAtomicUnit=on
  MATLAB Function3 : MATLAB Function  TreatAsAtomicUnit=on
  Moving Standard Deviation : dspstat3/Moving Standard Deviation  Method=Sliding window  ForgettingFactorPort=off  SpecifyWindowLength=on  WindowLength=g_standdev_window_size  OverlapLength=g_standdev_window_size-1  AllowArbitraryInputLength=off  ForgettingFactor=0.9  SimulateUsing=Code generation
  Sum : Sum  Inputs=|+-
  isDeviated : Outport
  likelihood : Outport  Port=2
  wires:
  Moving Standard Deviation/1 -> MATLAB Function/3(std_dev)
  MATLAB Function/1(likelihood) -> likelihood/1, MATLAB Function1/2(prob)
  Simulated o2 value/1 -> Sum/2
  Constant/1 -> MATLAB Function/4(o2_prob_arraylen)
  Sensor o2 value/1 -> MATLAB Function2/2(input), Sum/1
  Sum/1 -> MATLAB Function3/2(input)
  MATLAB Function1/1(isDeviated) -> isDeviated/1
  Constant1/1 -> MATLAB Function1/3(thresh)
  Constant2/1 -> MATLAB Function1/4(thresh_count)
  dnr/1 -> MATLAB Function2/1(DNR), MATLAB Function3/1(DNR), MATLAB Function/1(dnr), MATLAB Function1/1(dnr)
  MATLAB Function2/1(output) -> Moving Standard Deviation/1
  MATLAB Function3/1(output) -> MATLAB Function/2(new_sens_value)

== system digital_twin_model_v2/Attack and Fault Detection System/Oxygen Sensor Failure Detection ==
  o2_sensor : Inport
  dnr : Inport  Port=2
  Constant : Constant  Value=o2_fail_mean
  Constant2 : Constant  Value=o2_fault_halfrange
  Constant3 : Constant  Value=o2_fault_numpoints
  MATLAB Function2 : MATLAB Function  TreatAsAtomicUnit=on
  isFailed : Outport
  wires:
  Constant2/1 -> MATLAB Function2/4(half_range)
  Constant3/1 -> MATLAB Function2/5(num_points)
  Constant/1 -> MATLAB Function2/3(fail_val)
  o2_sensor/1 -> MATLAB Function2/2(o2_sensor)
  MATLAB Function2/1(isFailed) -> isFailed/1
  dnr/1 -> MATLAB Function2/1(dnr)

== system digital_twin_model_v2/Attack and Fault Detection System/Recycle Pump Fault Detection ==
  oxygen sensor : Inport
  dnr : Inport  Port=2
  net flowrate commanded : Inport  Port=3
  Constant : Constant  Value=recPump_drop_val
  Constant3 : Constant  Value=recPump_rollingavg_samples_buildup
  Constant4 : Constant  Value=recPump_smallDrop_size
  MATLAB Function : MATLAB Function  TreatAsAtomicUnit=on
  noRecycleResponse : Outport
  large drop : Outport  Port=2
  wires:
  net flowrate commanded/1 -> MATLAB Function/2(new_flowrate_commanded)
  MATLAB Function/1(RecyclePumpFail) -> noRecycleResponse/1
  oxygen sensor/1 -> MATLAB Function/3(oxygen_sensor)
  Constant/1 -> MATLAB Function/6(large_drop_val)
  Constant4/1 -> MATLAB Function/5(o2_rollavg_drop_spec)
  Constant3/1 -> MATLAB Function/4(samples_to_wait)
  dnr/1 -> MATLAB Function/1(dnr)
  MATLAB Function/2(largeDrop) -> large drop/1

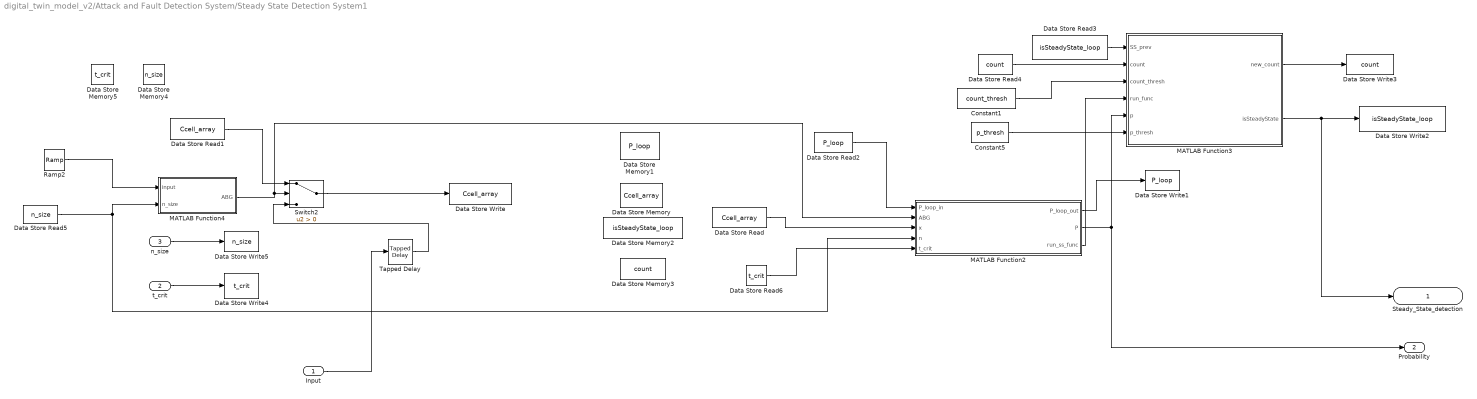
== system digital_twin_model_v2/Attack and Fault Detection System/Steady State Detection System1 ==
  Input : Inport
  t_crit : Inport  Port=2
  n_size : Inport  Port=3
  Constant1 : Constant  Value=count_thresh
  Constant5 : Constant  Value=p_thresh
  Data Store Memory : DataStoreMemory  DataStoreName=Ccell_array  ReadBeforeWriteMsg=warning  WriteAfterWriteMsg=warning  WriteAfterReadMsg=warning  InitialValue=zeros(1,n_size)  ShowAdditionalParam=off  OutDataTypeStr=double
  Data Store Memory1 : DataStoreMemory  DataStoreName=P_loop  ReadBeforeWriteMsg=warning  WriteAfterWriteMsg=warning  WriteAfterReadMsg=warning  ShowAdditionalParam=off
  Data Store Memory2 : DataStoreMemory  DataStoreName=isSteadyState_loop  ReadBeforeWriteMsg=warning  WriteAfterWriteMsg=warning  WriteAfterReadMsg=warning  ShowAdditionalParam=off
  Data Store Memory3 : DataStoreMemory  DataStoreName=count  ReadBeforeWriteMsg=warning  WriteAfterWriteMsg=warning  WriteAfterReadMsg=warning  ShowAdditionalParam=off
  Data Store Memory4 : DataStoreMemory  DataStoreName=n_size  ReadBeforeWriteMsg=warning  WriteAfterWriteMsg=warning  WriteAfterReadMsg=warning  ShowAdditionalParam=off
  Data Store Memory5 : DataStoreMemory  DataStoreName=t_crit  ReadBeforeWriteMsg=warning  WriteAfterWriteMsg=warning  WriteAfterReadMsg=warning  ShowAdditionalParam=off
  Data Store Read : DataStoreRead  DataStoreName=Ccell_array  IndexOptions=Index vector (dialog)  Indices=1  OutputSizes=1
  Data Store Read1 : DataStoreRead  DataStoreName=Ccell_array  IndexOptions=Index vector (dialog)  Indices=1  OutputSizes=1
  Data Store Read2 : DataStoreRead  DataStoreName=P_loop  IndexOptions=Index vector (dialog)  Indices=1  OutputSizes=1
  Data Store Read3 : DataStoreRead  DataStoreName=isSteadyState_loop  IndexOptions=Index vector (dialog)  Indices=1  OutputSizes=1
  Data Store Read4 : DataStoreRead  DataStoreName=count  IndexOptions=Index vector (dialog)  Indices=1  OutputSizes=1
  Data Store Read5 : DataStoreRead  DataStoreName=n_size  IndexOptions=Index vector (dialog)  Indices=1  OutputSizes=1
  Data Store Read6 : DataStoreRead  DataStoreName=t_crit  IndexOptions=Index vector (dialog)  Indices=1  OutputSizes=1
  Data Store Write : DataStoreWrite  DataStoreName=Ccell_array  IndexOptions=Index vector (dialog)  Indices=1  OutputSizes=1
  Data Store Write1 : DataStoreWrite  DataStoreName=P_loop  IndexOptions=Index vector (dialog)  Indices=1  OutputSizes=1
  Data Store Write2 : DataStoreWrite  DataStoreName=isSteadyState_loop  IndexOptions=Index vector (dialog)  Indices=1  OutputSizes=1
  Data Store Write3 : DataStoreWrite  DataStoreName=count  IndexOptions=Index vector (dialog)  Indices=1  OutputSizes=1
  Data Store Write4 : DataStoreWrite  DataStoreName=t_crit  IndexOptions=Index vector (dialog)  Indices=1  OutputSizes=1
  Data Store Write5 : DataStoreWrite  DataStoreName=n_size  IndexOptions=Index vector (dialog)  Indices=1  OutputSizes=1
  MATLAB Function2 : MATLAB Function  TreatAsAtomicUnit=on
  MATLAB Function3 : MATLAB Function  TreatAsAtomicUnit=on
  MATLAB Function4 : MATLAB Function  TreatAsAtomicUnit=on
  Ramp2 : simulink/Sources/Ramp  slope=1/ts  start=0  InitialOutput=0
  Switch2 : Switch  Criteria=u2 > Threshold  SaturateOnIntegerOverflow=off  InputSameDT=off
  Tapped Delay : simulink/Discrete/Tapped Delay  vinit=0.0  samptime=-1  NumDelays=n_size  DelayOrder=Oldest  includeCurrent=off
  Steady_State_detection : Outport
  Probability : Outport  Port=2
  wires:
  MATLAB Function3/2(isSteadyState) -> Steady_State_detection/1, Data Store Write2/1
  MATLAB Function2/1(P_loop_out) -> Data Store Write1/1
  Data Store Read2/1 -> MATLAB Function2/1(P_loop_in)
  Input/1 -> Tapped Delay/1
  Data Store Read4/1 -> MATLAB Function3/2(count)
  Data Store Read1/1 -> Switch2/1
  MATLAB Function2/2(P) -> Probability/1, MATLAB Function3/5(p)
  Constant5/1 -> MATLAB Function3/6(p_thresh)
  Data Store Read5/1 -> MATLAB Function4/2(n_size), MATLAB Function2/4(n)
  MATLAB Function3/1(new_count) -> Data Store Write3/1
  Ramp2/1 -> MATLAB Function4/1(input)
  MATLAB Function4/1(ABG) -> MATLAB Function2/2(ABG), Switch2/2
  Tapped Delay/1 -> Switch2/3
  Data Store Read6/1 -> MATLAB Function2/5(t_crit)
  t_crit/1 -> Data Store Write4/1
  n_size/1 -> Data Store Write5/1
  Data Store Read/1 -> MATLAB Function2/3(x)
  Switch2/1 -> Data Store Write/1
  MATLAB Function2/3(run_ss_func) -> MATLAB Function3/4(run_func)
  Data Store Read3/1 -> MATLAB Function3/1(SS_prev)
  Constant1/1 -> MATLAB Function3/3(count_thresh)

== matlab function digital_twin_model_v2/Subsystem/MATLAB Function1 ==
  data: reactor_dnr input; detection_dnr output; change_detected input
function detection_dnr = fcn(reactor_dnr, change_detected)

persistent flag2;

if isempty(flag2)
    flag2=0;
end

if reactor_dnr==1
    detection_dnr=1;
else
    if change_detected==true
        detection_dnr=0;
        flag2=0;
    else %change_detected==false
        if flag2==1
            detection_dnr=1;
        else %flag2==0
            detection_dnr=0;
            flag2=1;
        end
    end
end

== matlab function digital_twin_model_v2/Digital Reactor/maintain previous CG and Co values if DNR is true ==
  data: oldCG input; CG_out output; newCG input; oldCO input; newCO input; oldCcell input; newCcell input; doNotRun input; CO_out output; Ccell_out output
function [CG_out, CO_out, Ccell_out] = noChange(oldCG, newCG, oldCO, newCO, oldCcell, newCcell, doNotRun)

if doNotRun==1
    CG_out = oldCG;
    CO_out = oldCO;
    Ccell_out = oldCcell;
else %doNotRUn==0
    CG_out = newCG;
    CO_out = newCO;
    Ccell_out = newCcell;
end

== matlab function digital_twin_model_v2/Attack and Fault Detection System/Glucose Deviation Detection/MATLAB Function2 ==
  data: DNR input; output output; input input
function output = echoIfDNR(DNR, input)

persistent lastInput3;

if isempty(lastInput3)
    lastInput3=0;
end

if DNR==1
    output = lastInput3;
else %DNR==0
    output = input;
    lastInput3 = input;
end

== matlab function digital_twin_model_v2/Attack and Fault Detection System/Glucose Deviation Detection/MATLAB Function3 ==
  data: DNR input; output output; input input
function output = echoIfDNR(DNR, input)

persistent lastInput4;

if isempty(lastInput4)
    lastInput4=0;
end

if DNR==1
    output = lastInput4;
else %DNR==0
    output = input;
    lastInput4 = input;
end

== matlab function digital_twin_model_v2/Attack and Fault Detection System/Glucose Fault Detection/MATLAB Function1 ==
  data: DNR input; output output; input input
function output = echoIfDNR(DNR, input)

persistent lastInput6;

if isempty(lastInput6)
    lastInput6=0;
end

if DNR==1
    output = lastInput6;
else %DNR==0
    output = input;
    lastInput6 = input;
end

== matlab function digital_twin_model_v2/Digital Reactor/MATLAB Function ==
  data: mu_max input; CM input; CG input; Ccell input; cgNoGrowth input; dCcell_dt output; ts input; CO input; dnr input
function dCcell_dt  = monodEq(mu_max, CM,CG,Ccell, cgNoGrowth, ts, CO, dnr) %,volume, cgNo)


dCcell_dt = (mu_max * Ccell * CG) / (CG + CM) * ts;

if (dCcell_dt < 0 || CG<=cgNoGrowth || CO<=.01 || dnr==1)
    dCcell_dt = 0;
end

%val = (CG * volume / 100) / Ccell;

%if (val < cgNo)
%    dCcell_dt = 0;
%end

== matlab function digital_twin_model_v2/Attack and Fault Detection System/Oxygen Deviation Detection1/MATLAB Function2 ==
  data: DNR input; output output; input input
function output = echoIfDNR(DNR, input)

persistent lastInput7;

if isempty(lastInput7)
    lastInput7=0;
end

if DNR==1
    output = lastInput7;
else %DNR==0
    output = input;
    lastInput7 = input;
end

== matlab function digital_twin_model_v2/Attack and Fault Detection System/Oxygen Deviation Detection1/MATLAB Function3 ==
  data: DNR input; output output; input input
function output = echoIfDNR(DNR, input)

persistent lastInput8;

if isempty(lastInput8)
    lastInput8=0;
end

if DNR==1
    output = lastInput8;
else %DNR==0
    output = input;
    lastInput8 = input;
end

== matlab function digital_twin_model_v2/Subsystem1/MATLAB Function ==
  data: code1 input; fullCode output; code2 input; code3 input; code4 input; code5 input; code6 input; code7 input
function fullCode  = faultCode(code1, code2, code3, code4, code5, code6, code7)


%combine into array
inputs = [code1, code2, code3, code4, code5, code6, code7];

sortedInputs = sort(inputs);

% Remove zeros
nonZeroInputs = sortedInputs(sortedInputs ~= 0);

% Convert the array to a single number without using str2num
fullCode = 0;
for i = 1:length(nonZeroInputs)
    fullCode = fullCode * 10 + nonZeroInputs(i);
end

== matlab function digital_twin_model_v2/Digital Reactor/MATLAB Function1 ==
  data: in input; out output
function out = notZero(in)

if in>0
    out=in;
else % in<0
    out = 0;
end

== matlab function digital_twin_model_v2/Attack and Fault Detection System/Glucose Abnormally Low Noise Detection/MATLAB Function3 ==
  data: dnr input; noiseSmall output; stdev_sensor input; stdev_tol input; num_points input; ignore_over input
function noiseSmall = detectGFailure(dnr, stdev_sensor, stdev_tol, num_points, ignore_over)

%create fail count variable
persistent count_g_low;
%fill it if full
if isempty(count_g_low)
    count_g_low = 0;
end

if (dnr==0)
    if count_g_low==num_points
        noiseSmall = 1;
    else
        if (stdev_sensor<=stdev_tol && ignore_over == 1)
            count_g_low = count_g_low + 1;
        else
            count_g_low = 0;
        end
        noiseSmall = 0;
    end
else
    noiseSmall=0;
end
